simulink model "Robot_calibration_check_Ipos"  (R2021a)
settings: Solver=FixedStepDiscrete  StartTime=0.0  StopTime=tsim  FixedStep=Ts  RelTol=1e-3  EnableMultiTasking=on
InitFcn:
  | Fs = 2048; Ts = 1/Fs;tsim = inf;
undefined symbols (not defined in the file or in its folder): DiscIntNeverNeededParam
libraries: sperte_lib x24, simulink x6, raspberrypiCommlib x2, Quintic_Polynomial_Trajectory_Library x2
(part 1 of 2)
settings Model: SimulationMode=external  Creator=20174295  LastModifiedBy=ghattum
settings SolverCC: AlgebraicLoopSolver=TrustRegion  PositivePriorityOrder=on
settings DataIOCC: SaveOutput=off  DSMLogging=off  SaveTime=off  ReturnWorkspaceOutputs=off
settings OptimizationCC: EnhancedBackFolding=on  PassReuseOutputArgsThreshold=0  MaxStackSize=64  OptimizeBlockOrder=speed  DifferentSizesBufferReuse=on  OptimizationCustomize=off
settings DebuggingCC: InheritedTsInSrcMsg=none  ParameterTunabilityLossMsg=error  SFMachineParentedDataDiag=warning
settings HardwareCC: ProdBitPerPointer=32  ProdBitPerSizeT=32  ProdBitPerPtrDiffT=32  ProdLargestAtomicInteger=Long  ProdLargestAtomicFloat=Double  ProdWordSize=32  ProdLongLongMode=on  ProdHWDeviceType=ARM Compatible->ARM Cortex  UseEmbeddedCoderFeatures=off
settings RTWCC: SystemTargetFile=ert.tlc  HardwareBoard=Raspberry Pi  TLCOptions="-aInlineSetEventsForThisBaseRateFcn=TLC_FALSE -aSuppressMultiTaskScheduler=TLC_FALSE  -aRateBasedStepFcn=0"  TemplateMakefile=ert_default_tmf  PostCodeGenCommand="if (~verLessThan(\"matlab\", \"9.11\")) codertarget.postCodeGenHookCommand(h);  SPERTE_postGenFunc(modelName, buildInfo); else; SPERTE_postGenFunc(h, buildInfo); end"  Toolchain=GNU GCC Embedded Linux  BuildConfiguration=Faster Runs
settings CodeAppCC: ForceParamTrailComments=on  OperatorAnnotations=on
settings ERTTargetCC: ERTCustomFileBanners=off  SupportContinuousTime=on  SupportNonInlinedSFcns=on  RemoveResetFunc=off  SupportVariableSizeSignals=on  ModelStepFunctionPrototypeControlCompliant=off  ExtMode=on  ExtModeStaticAlloc=on  ExtModeMexArgs='10.55.0.1' 0 17726  ERTSrcFileBannerTemplate=codertarget_code_template.cgt  ERTHdrFileBannerTemplate=codertarget_code_template.cgt  ERTDataSrcFileTemplate=codertarget_code_template.cgt  ERTDataHdrFileTemplate=codertarget_code_template.cgt

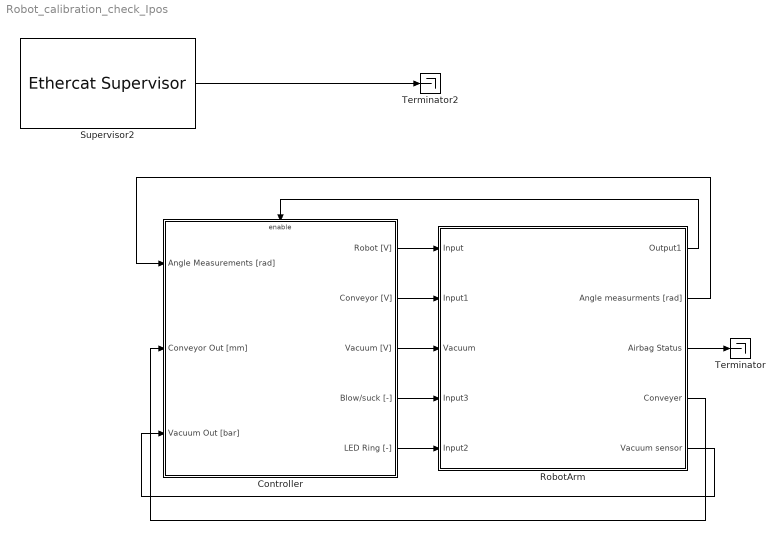
== system Robot_calibration_check_Ipos ==
  Controller : Subsystem
  RobotArm : Subsystem
      mask help:
      | Robot Arm
      | Hardware: Brom Mechatronica
      | Software: Bob Bindels, Victor Dolk, Quinten Swaan, Hugo Thelosen
      mask Display:
      | image(imread('picture_robot.jpg'))
      | color('red');port_label('output', 1, 'Homing Busy [-]')
      | port_label('output', 2, 'Angle Measurements [rad]')
      | port_label('output', 3, 'Airbag Status [-]')
      | port_label('output', 4, 'Conveyor Belt [mm]')
      | port_label('output', 5, 'Vacuum Sensor [bar]')
      | port_label('input', 1, 'Input Robot [V]')
      | port_label('input', 2,'Input Conv [V]' )
      | port_label('input', 3,'Input Vac [V]' )
      | port_label('input', 4,'IO Vac [-]' )
      | port_label('input', 5,'LED-Ring [-]' )
  Supervisor2 : sperte_lib/Ethercat Supervisor  Description=Must be executed first, keep at -1 priority (highest)  Priority=-3  portid=0  ectimeout=500
      settings: SourceProductName=SPERTE project library
  Terminator : Terminator
  Terminator2 : Terminator
  wires:
  Supervisor2/1 -> Terminator2/1
  Controller/1(Robot [V]) -> RobotArm/1(Input)
  RobotArm/1(Output1) -> Controller/Enable
  RobotArm/2(Angle measurments [rad]) -> Controller/1(Angle Measurements [rad])
  Controller/2("Conveyor [V] ") -> RobotArm/2(Input1)
  Controller/3("Vacuum [V] ") -> RobotArm/3(Vacuum)
  Controller/4(Blow/suck [-]) -> RobotArm/4(Input3)
  RobotArm/3(Airbag Status) -> Terminator/1
  RobotArm/4(Conveyer) -> Controller/2(Conveyor Out [mm])
  Controller/5(LED Ring [-]) -> RobotArm/5(Input2)
  RobotArm/5(Vacuum sensor) -> Controller/3(Vacuum Out [bar])

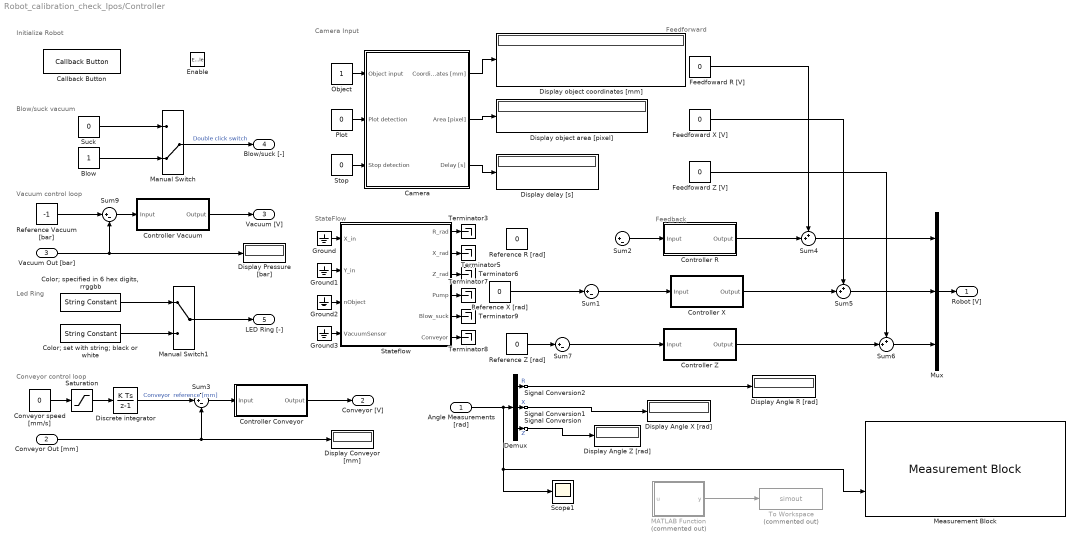
== system Robot_calibration_check_Ipos/Controller ==
  note: Feedforward
  note: StateFlow
  note: Camera Input
  note: Vacuum control loop
  note: Conveyor control loop
  note: Blow/suck vacuum
  note: Led Ring
  note: Feedback
  note: Initialize Robot
  Angle Measurements [rad] : Inport
  Conveyor Out [mm] : Inport  Port=2
  Vacuum Out [bar] : Inport  Port=3
  "Enable " : EnablePort
  " Blow" : Constant
  Callback Button : CallbackButton  ButtonText=INITIALIZE MODEL
      settings: ClickFcn=|
      | robot_number = input('What is your Robot number?: ');
      | file_name_simulink = get_param(bdroot, 'Name');
      | load('calibration_matrix.mat');
      | [camera_calibration_x_pixels,camera_calibration_y_pixels,camera_calibration_pixels_per_mm,camera_calibration_ROI,robot_calibration_r,robot_calibration_x, robot_calibration_z] = Calibrate_Robot_Settings(robot_number,calibration)
      | 
      | set_param(file_name_simulink+"/RobotArm/Supervisor/set_robot_calibration_r",'Value',num2str(robot_calibration_r));
      | set_param(file_name_simulink+"/RobotArm/Supervisor/set_robot_calibration_x",'Value',num2str(robot_calibration_x));
      | set_param(file_name_simulink+"/RobotArm/Supervisor/set_robot_calibration_z",'Value',num2str(robot_calibration_z));
      | 
      | % robot_calibration_r = eval(get_param(file_name_simulink+"/RobotArm/Supervisor/set_robot_calibration_r",'Value'));
      | % robot_calibration_x = eval(get_param(file_name_simulink+"/RobotArm/Supervisor/set_robot_calibration_x",'Value'));
      | % robot_calibration_z = eval(get_param(file_name_simulink+"/RobotArm/Supervisor/set_robot_calibration_z",'Value'));
      | 
      | clear calibration
      | msgbox('Successfully initialized the model.');
  Camera : Subsystem
  Color; set with string; black or white : StringConstant  String='black'
  "Color; specified in 6 hex digits, rrggbb" : StringConstant  String='0072bd'
  Controller Conveyor : Subsystem
  Controller R : Subsystem
  Controller Vacuum : Subsystem
  Controller X : Subsystem
  Controller Z : Subsystem
  Conveyor speed [mm/s] : Constant  Value=0
  Demux : Demux  Outputs=3
  Discrete integrator : DiscreteIntegrator  SampleTime=-1  ICPrevOutput=DiscIntNeverNeededParam  ICPrevScaledInput=DiscIntNeverNeededParam
  Display Angle R [rad] : Display
  Display Angle X [rad] : Display
  Display Angle Z [rad] : Display
  Display Conveyor [mm] : Display
  Display Pressure [bar] : Display
  Display delay [s] : Display
  Display object area [pixel] : Display
  Display object coordinates [mm] : Display
  Feedfoward R [V] : Constant  Value=0
  Feedfoward X [V] : Constant  Value=0
  Feedfoward Z [V] : Constant  Value=0
  Ground{,1..3} (4 alike) : Ground
  MATLAB Function : MATLAB Function  Commented=on  TreatAsAtomicUnit=on
  Manual Switch : ManualSwitch  CurrentSetting=0
  Manual Switch1 : ManualSwitch
  Measurement Block : sperte_lib/Measurement Block  Description=|  Priority=-1  N_samples=1  triggertype=1  trigger_command=0
      | Perform on-demand measurements to file using this block.
      | 
      | It can be used in 2 ways:
      | 1) Set the mask triggertype parameter to manual and use the trigger input signal to trigger a measurement.
      | You can do this by providing a 0 to 1 transition.
      | Keep it low after you start/complete the measurement, or it will measure again.
      | A file is created with measurement_0,1,2... etc
      | 
      | 2) Keep the model running, and trigger a measurement from the commandline or Matlab script.
      | For example:
      | 
      | % How many samples to measure?
      | N_samples = Fs*5;
      | % Do the measurement
      | SPERTE_Perform_Measurement(N_samples);
      | % Get the latest file
      | file_list = SPERTE_Get_Latest_Measurement(p,1,'./data');
      | % How many signals did you record?
      | N_signals = 3;
      | % Convert the .bin to .mat and return the results
      | measurement = SPERTE_Bin_To_Mat(file_list,N_signals);
      settings: SourceProductName=SPERTE project library
  Mux : Mux  Inputs=3
  Object : Constant
  Plot : Constant  Value=0
  Reference Vacuum [bar] : Constant  Value=-1
  Reference R [rad] : Constant  Value=0
  Reference X [rad] : Constant  Value=0
  Reference Z [rad] : Constant  Value=0
  "Saturation " : Saturate  UpperLimit=100  LowerLimit=-100
  Scope1 : Scope
  Signal Conversion : SignalConversion  OverrideOpt=off
  Signal Conversion1 : SignalConversion  OverrideOpt=off
  Signal Conversion2 : SignalConversion  OverrideOpt=off
  "Stateflow " : Stateflow chart  TreatAsAtomicUnit=on
  Stop : Constant  Value=0
  Suck : Constant  Value=0
  Sum{1..3,7,9} (5 alike) : Sum  Inputs=|+-
  Sum4 : Sum  Inputs=++|  InputSameDT=on  SaturateOnIntegerOverflow=on  OutDataTypeStr=Inherit: Same as first input
  Sum5 : Sum  Inputs=++|  InputSameDT=on  SaturateOnIntegerOverflow=on  OutDataTypeStr=Inherit: Same as first input
  Sum6 : Sum  Inputs=++|  InputSameDT=on  SaturateOnIntegerOverflow=on  OutDataTypeStr=Inherit: Same as first input
  Terminator{3,5..9} (6 alike) : Terminator
  To Workspace : ToWorkspace  Commented=on  VariableName=simout  SaveFormat=Timeseries  SampleTime=-1
  Robot [V] : Outport
  "Conveyor [V] " : Outport  Port=2
  "Vacuum [V] " : Outport  Port=3
  Blow/suck [-] : Outport  Port=4
  LED Ring [-] : Outport  Port=5
  wires:
  Manual Switch/1 -> Blow/suck [-]/1  "Double click switch"
  Suck/1 -> Manual Switch/1
  " Blow"/1 -> Manual Switch/2
  Feedfoward Z [V]/1 -> Sum6/1
  Sum7/1 -> Controller Z/1(Input)
  Controller Z/1(Output) -> Sum6/2
  Controller X/1(Output) -> Sum5/2
  Controller R/1(Output) -> Sum4/2
  Demux/2 -> Signal Conversion1/1  "X"
  Mux/1 -> Robot [V]/1
  Demux/3 -> Signal Conversion/1  "Z"
  Angle Measurements [rad]/1 -> Measurement Block/2, Scope1/1, Demux/1
  "Color; specified in 6 hex digits, rrggbb"/1 -> Manual Switch1/1
  Color; set with string; black or white/1 -> Manual Switch1/2
  Demux/1 -> Signal Conversion2/1  "R"
  Manual Switch1/1 -> LED Ring [-]/1
  Vacuum Out [bar]/1 -> Sum9/2, Display Pressure [bar]/1
  Sum1/1 -> Controller X/1(Input)
  Stop/1 -> Camera/3(Stop detection)
  Object/1 -> Camera/1(Object input)
  Plot/1 -> Camera/2(Plot detection)
  Reference Vacuum [bar]/1 -> Sum9/1
  Sum9/1 -> Controller Vacuum/1(Input)
  Controller Vacuum/1(Output) -> "Vacuum [V] "/1
  Signal Conversion/1 -> Display Angle Z [rad]/1
  Signal Conversion1/1 -> Display Angle X [rad]/1
  Signal Conversion2/1 -> Display Angle R [rad]/1
  Ground/1 -> "Stateflow "/1(X_in)
  Ground1/1 -> "Stateflow "/2(Y_in)
  Ground2/1 -> "Stateflow "/3(nObject)
  Ground3/1 -> "Stateflow "/4(VacuumSensor)
  "Stateflow "/1(R_rad) -> Terminator3/1
  "Stateflow "/2(X_rad) -> Terminator5/1
  "Stateflow "/3(Z_rad) -> Terminator6/1
  "Stateflow "/4(Pump) -> Terminator7/1
  "Stateflow "/5(Blow_suck) -> Terminator9/1
  "Stateflow "/6(Conveyor) -> Terminator8/1
  Discrete integrator/1 -> Sum3/1  "Conveyor  reference [mm]"
  Conveyor speed [mm/s]/1 -> "Saturation "/1
  "Saturation "/1 -> Discrete integrator/1
  Camera/1(Coordinates [mm]) -> Display object coordinates [mm]/1
  Camera/3(Delay [s]) -> Display delay [s]/1
  Camera/2(Area [pixel]) -> Display object area [pixel]/1
  Sum6/1 -> Mux/3
  Controller Conveyor/1(Output) -> "Conveyor [V] "/1
  Sum4/1 -> Mux/1
  Sum2/1 -> Controller R/1(Input)
  Reference Z [rad]/1 -> Sum7/1
  Feedfoward X [V]/1 -> Sum5/1
  Sum5/1 -> Mux/2
  Reference X [rad]/1 -> Sum1/1
  Feedfoward R [V]/1 -> Sum4/1
  Conveyor Out [mm]/1 -> Display Conveyor [mm]/1, Sum3/2
  Sum3/1 -> Controller Conveyor/1(Input)
  MATLAB Function/1(y) -> To Workspace/1

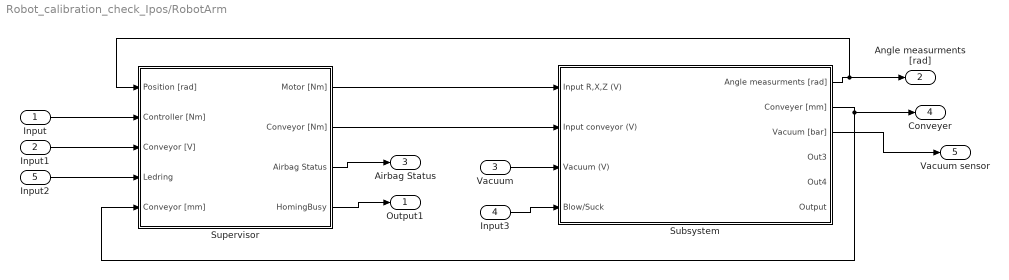
== system Robot_calibration_check_Ipos/RobotArm ==
  Input : Inport
  Input1 : Inport  Port=2
  Vacuum : Inport  Port=3
  Input3 : Inport  Port=4
  Input2 : Inport  Port=5
  Subsystem : Subsystem
  Supervisor : Subsystem
  Output1 : Outport
  Angle measurments [rad] : Outport  Port=2
  Airbag Status : Outport  Port=3
  Conveyer : Outport  Port=4
  Vacuum sensor : Outport  Port=5
  wires:
  Supervisor/1(Motor [Nm]) -> Subsystem/1(Input R,X,Z (V))
  Subsystem/2(Conveyer [mm]) -> Supervisor/5(Conveyor [mm]), Conveyer/1
  Supervisor/4(HomingBusy) -> Output1/1
  Input/1 -> Supervisor/2(Controller [Nm])
  Subsystem/1(Angle measurments [rad]) -> Supervisor/1(Position [rad]), Angle measurments [rad]/1
  Input1/1 -> Supervisor/3(Conveyor [V])
  Input3/1 -> Subsystem/4(Blow/Suck)
  Supervisor/3(Airbag Status) -> Airbag Status/1
  Supervisor/2(Conveyor [Nm]) -> Subsystem/2(Input conveyor (V))
  Input2/1 -> Supervisor/4(Ledring)
  Subsystem/3(Vacuum [bar]) -> Vacuum sensor/1
  Vacuum/1 -> Subsystem/3(Vacuum (V))

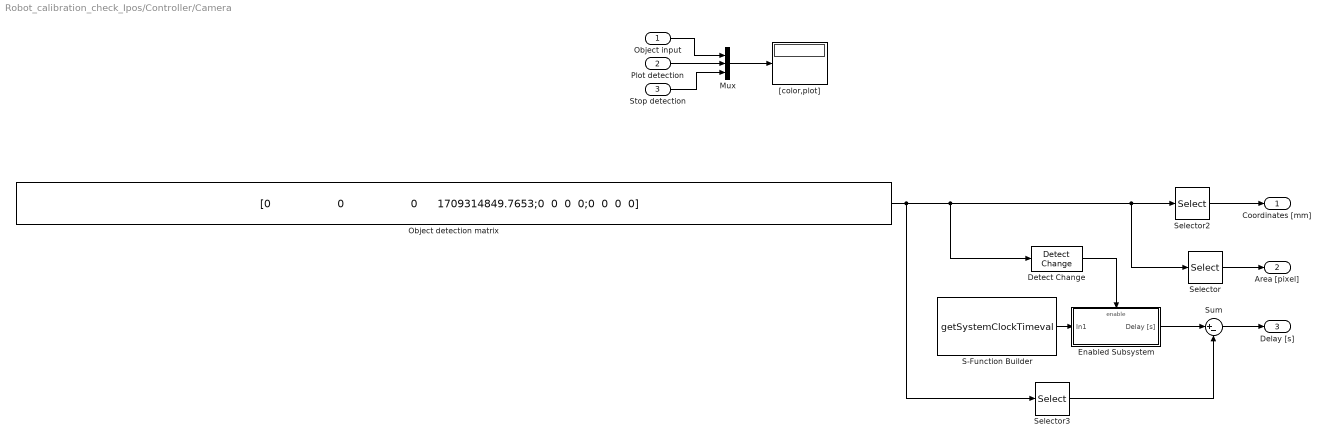
== system Robot_calibration_check_Ipos/Controller/Camera ==
  Object input : Inport
  Plot detection : Inport  Port=2
  Stop detection : Inport  Port=3
  Detect Change : simulink/Logic and Bit Operations/Detect Change  vinit=0  OutDataTypeStr=boolean
  Enabled Subsystem : Subsystem  TreatAsAtomicUnit=on
  Mux : Mux  Inputs=3
  Object detection matrix : Constant  Value="[0                    0                    0      1709314849.7653;0  0  0  0;0  0  0  0]"  VectorParams1D=off
  S-Function Builder : S-Function  InitFcn=try, set_param(gcb,'FunctionName','getSystemClockTimeval'), end  FunctionName=getSystemClockTimeval  SFunctionModules=getSystemClockTimeval_wrapper  SFunctionDeploymentMode=off  EnableBusSupport=off  mask(S-Function Builder){}
      mask help: Simulink:masks:SFunctionBuilder_MD
      mask init:
      | val = [[.9  0.75 0.75 1 1 .9 .9 1]',[1 1 0.75 0.75 .9 .9 1 .9]'];try , sys = get_param(gcb,'SfunBuilderFcnName');if isempty(sys), sys = get_param(gcb,'FunctionName'); end,catch, sys = get_param(gcb,'FunctionName'); end
      settings: CopyFcn=set_param(gcbh,'LinkStatus','none')  PreSaveFcn=try, set_param(gcb,'FunctionName','getSystemClockTimeval'), end  OpenFcn=sfunctionwizard(gcbh)
      mask Display: plot(val(:,1),val(:,2)),disp(sys),port_label('output',1,'y2')
  Selector : Selector  NumberOfDimensions=2  InputPortWidth=3  IndexOptions=Index vector (dialog),Index vector (dialog)  Indices=[3],[1:3]  OutputSizes=1,1
  Selector2 : Selector  NumberOfDimensions=2  InputPortWidth=3  IndexOptions=Select all,Index vector (dialog)  Indices=1,[1:3]  OutputSizes=1,1
  Selector3 : Selector  NumberOfDimensions=2  InputPortWidth=3  IndexOptions=Index vector (dialog),Index vector (dialog)  Indices=1,4  OutputSizes=1,1
  Sum : Sum  Inputs=|+-
  "[color,plot]" : Display
  Coordinates [mm] : Outport
  Area [pixel] : Outport  Port=2
  Delay [s] : Outport  Port=3
  wires:
  Object input/1 -> Mux/1
  Plot detection/1 -> Mux/2
  Mux/1 -> "[color,plot]"/1
  Stop detection/1 -> Mux/3
  Selector2/1 -> Coordinates [mm]/1
  Object detection matrix/1 -> Selector3/1, Detect Change/1, Selector/1, Selector2/1
  Detect Change/1 -> Enabled Subsystem/Enable
  S-Function Builder/1 -> Enabled Subsystem/1(In1)
  Enabled Subsystem/1(Delay [s]) -> Sum/1
  Sum/1 -> Delay [s]/1
  Selector3/1 -> Sum/2
  Selector/1 -> Area [pixel]/1

== system Robot_calibration_check_Ipos/Controller/Controller Conveyor ==
  Input : Inport
  Dct1lowpass : sperte_lib/Dct1lowpass  f_den=40
      settings: SourceProductName=SPERTE project library
  Dctintegrator3 : S-Function  FunctionName=dweakint  Parameters=f_num, 0.001  SFunctionDeploymentMode=off  EnableBusSupport=off  mask(dctools){f_num=0.05}
      mask prompts: f_num "Zero [Hz]"
      mask help: This block implements a discrete time weak integrator filter.
      mask Display: disp('DCT integrator')
  Dctleadlag : sperte_lib/Dctleadlag  f_num=3  f_den=30
      settings: SourceProductName=SPERTE project library
  Gain1 : Gain  Gain=0.05
  Output : Outport
  wires:
  Input/1 -> Gain1/1
  Dctintegrator3/1 -> Dct1lowpass/1
  Dctleadlag/1 -> Output/1
  Gain1/1 -> Dctintegrator3/1
  Dct1lowpass/1 -> Dctleadlag/1

== system Robot_calibration_check_Ipos/Controller/Controller R ==
  Input : Inport
  Gain : Gain  Gain=5
  Output : Outport
  wires:
  Input/1 -> Gain/1
  Gain/1 -> Output/1

== system Robot_calibration_check_Ipos/Controller/Controller Vacuum ==
  Input : Inport
  Gain1 : Gain  Gain=-10
  Output : Outport
  wires:
  Input/1 -> Gain1/1
  Gain1/1 -> Output/1

== system Robot_calibration_check_Ipos/Controller/Controller X ==
  Input : Inport
  Gain1 : Gain  Gain=5
  Output : Outport
  wires:
  Gain1/1 -> Output/1
  Input/1 -> Gain1/1

== system Robot_calibration_check_Ipos/Controller/Controller Z ==
  Input : Inport
  Gain : Gain  Gain=5
  Output : Outport
  wires:
  Input/1 -> Gain/1
  Gain/1 -> Output/1

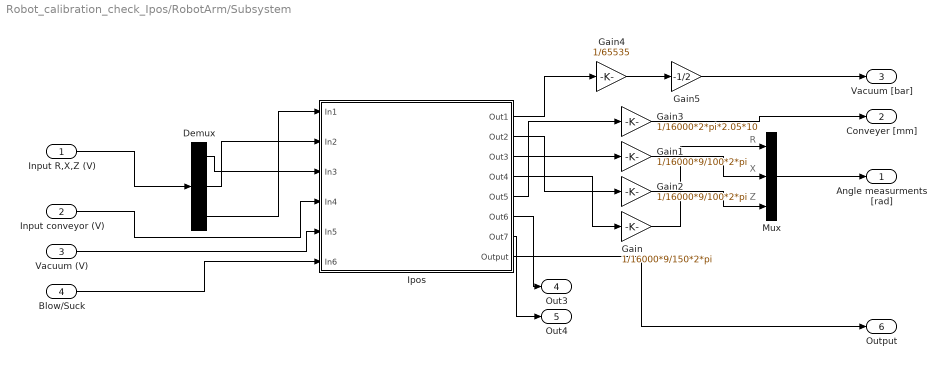
== system Robot_calibration_check_Ipos/RobotArm/Subsystem ==
  note: R
  note: X
  note: Z
  Input R,X,Z (V) : Inport
  Input conveyor (V) : Inport  Port=2
  Vacuum (V) : Inport  Port=3
  Blow/Suck : Inport  Port=4
  Demux : Demux  Outputs=3
  Gain : Gain  Gain=1/16000*9/150*2*pi
  Gain1 : Gain  Gain=1/16000*9/100*2*pi
  Gain2 : Gain  Gain=1/16000*9/100*2*pi
  Gain3 : Gain  Gain=1/16000*2*pi*2.05*10
  Gain4 : Gain  Gain=1/65535
  Gain5 : Gain  Gain=-1/2
  Ipos : Subsystem  mask{link_id=1}
      mask prompts: link_id "Link ID of the specific Ipos"
      mask Display:
      | image('ipos360.JPG'); % Use "Edit Image" on toolstrip to change.
      | port_label('output',1,'ADC')
      | port_label('output',2,'ENC1')
      | port_label('output',3,'ENC2')
      | port_label('output',4,'ENC3')
      | port_label('output',5,'ENC4')
      | port_label('output',6,'DI_t')
      | port_label('output',7,'DI_stop')
      | port_label('input',1,'Torque Conveyor')
      | port_label('input',2,'Torque X')
      | port_label('input',3,'Torque Z')
      | port_label('input',4,'Torque R')
      | port_label('input',5,'Do')
      | port_label('input',6,'setpoint_P')
  Mux : Mux  Inputs=3
  Angle measurments [rad] : Outport
  Conveyer [mm] : Outport  Port=2
  Vacuum [bar] : Outport  Port=3
  Out3 : Outport  Port=4
  Out4 : Outport  Port=5
  Output : Outport  Port=6
  wires:
  Mux/1 -> Angle measurments [rad]/1
  Input conveyor (V)/1 -> Ipos/4(In4)
  Ipos/8(Output) -> Output/1
  Gain1/1 -> Mux/2
  Input R,X,Z (V)/1 -> Demux/1
  Gain/1 -> Mux/1
  Ipos/7(Out7) -> Out4/1
  Gain2/1 -> Mux/3
  Gain3/1 -> Conveyer [mm]/1
  Ipos/1(Out1) -> Gain4/1
  Ipos/6(Out6) -> Out3/1
  Ipos/2(Out2) -> Gain2/1
  Ipos/3(Out3) -> Gain1/1
  Ipos/4(Out4) -> Gain/1
  Ipos/5(Out5) -> Gain3/1
  Demux/2 -> Ipos/2(In2)
  Demux/3 -> Ipos/1(In1)
  Blow/Suck/1 -> Ipos/6(In6)
  Vacuum (V)/1 -> Ipos/5(In5)
  Demux/1 -> Ipos/3(In3)
  Gain4/1 -> Gain5/1
  Gain5/1 -> Vacuum [bar]/1

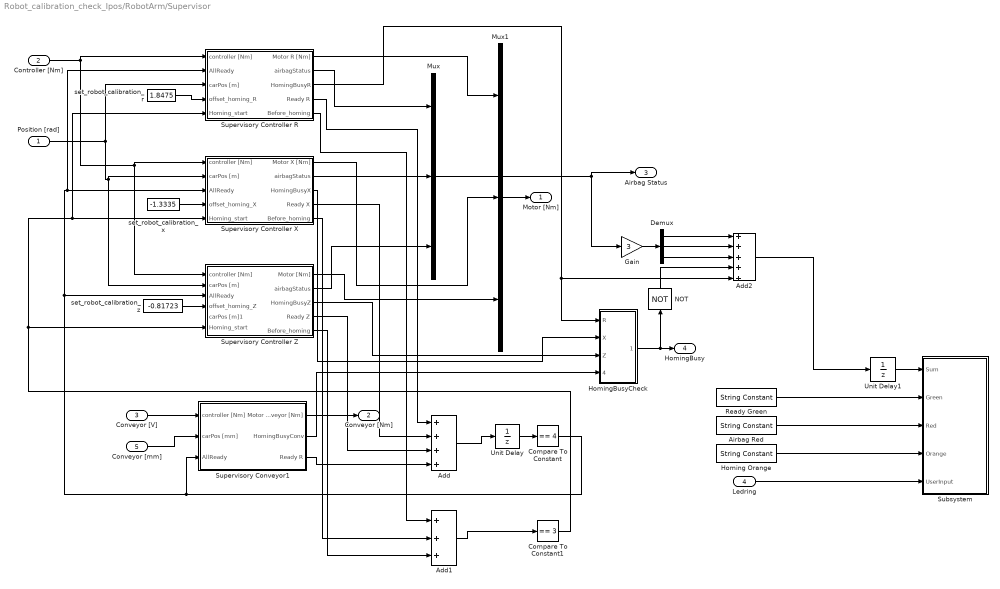
== system Robot_calibration_check_Ipos/RobotArm/Supervisor ==
  Position [rad] : Inport
  Controller [Nm] : Inport  Port=2
  Conveyor [V] : Inport  Port=3
  Ledring : Inport  Port=4
  Conveyor [mm] : Inport  Port=5
  Add : Sum  Inputs=++++
  Add1 : Sum  Inputs=+++
  Add2 : Sum  Inputs=+++++
  Airbag Red : StringConstant  String='00FF0000'
  Compare To Constant : simulink/Logic and Bit Operations/Compare To Constant  relop===  const=4  OutDataTypeStr=boolean
  Compare To Constant1 : simulink/Logic and Bit Operations/Compare To Constant  relop===  const=3  OutDataTypeStr=boolean
  Demux : Demux  Outputs=3
  Gain : Gain  Gain=3
  Homing Orange : StringConstant  String='00FF3900'
  HomingBusyCheck : Subsystem
  Mux : Mux  Inputs=3
  Mux1 : Mux  Inputs=3
  NOT : Logic  Operator=NOT  IconShape=distinctive  AllPortsSameDT=off  OutDataTypeStr=boolean
  Ready Green : StringConstant  String='0000FF00'
  Subsystem : Subsystem
  Supervisory Controller R : Subsystem
  Supervisory Controller X : Subsystem
  Supervisory Controller Z : Subsystem
  Supervisory Conveyor1 : Subsystem
  Unit Delay : UnitDelay  SampleTime=-1  HasFrameUpgradeWarning=on
  Unit Delay1 : UnitDelay  SampleTime=-1  HasFrameUpgradeWarning=on
  set_robot_calibration_r : Constant  Value=1.8475
  set_robot_calibration_x : Constant  Value=-1.3335
  set_robot_calibration_z : Constant  Value=-0.81723
  Motor [Nm] : Outport
  Conveyor [Nm] : Outport  Port=2
  Airbag Status : Outport  Port=3
  HomingBusy : Outport  Port=4
  wires:
  Controller [Nm]/1 -> Supervisory Controller R/1(controller [Nm]), Supervisory Controller X/1(controller [Nm]), Supervisory Controller Z/1(controller [Nm])
  Supervisory Controller R/2(airbagStatus) -> Mux/1
  Supervisory Controller X/2(airbagStatus) -> Mux/2
  Supervisory Controller Z/2(airbagStatus) -> Mux/3
  Position [rad]/1 -> Supervisory Controller R/3(carPos [m]), Supervisory Controller X/2(carPos [m]), Supervisory Controller Z/2(carPos [m])
  Mux1/1 -> Motor [Nm]/1
  Supervisory Controller X/3(HomingBusyX) -> HomingBusyCheck/2(X)
  Supervisory Controller Z/3(HomingBusyZ) -> HomingBusyCheck/3(Z)
  HomingBusyCheck/1(Out1) -> NOT/1, HomingBusy/1
  Supervisory Controller R/4(Ready R) -> Add/1
  Supervisory Controller X/4(Ready X) -> Add/2
  Supervisory Controller Z/4(Ready Z) -> Add/3
  Compare To Constant/1 -> Supervisory Controller X/3(AllReady), Supervisory Controller R/2(AllReady), Supervisory Controller Z/3(AllReady), Supervisory Conveyor1/3(AllReady)
  Add/1 -> Unit Delay/1
  Unit Delay/1 -> Compare To Constant/1
  set_robot_calibration_r/1 -> Supervisory Controller R/4(offset_homing_R)
  set_robot_calibration_x/1 -> Supervisory Controller X/4(offset_homing_X)
  set_robot_calibration_z/1 -> Supervisory Controller Z/4(offset_homing_Z)
  Mux/1 -> Airbag Status/1, Gain/1
  Supervisory Controller R/5(Before_homing) -> Add1/1
  Supervisory Controller X/5(Before_homing) -> Add1/2
  Supervisory Controller Z/5(Before_homing) -> Add1/3
  Add1/1 -> Compare To Constant1/1
  Compare To Constant1/1 -> Supervisory Controller Z/6(Homing_start), Supervisory Controller X/5(Homing_start), Supervisory Controller R/5(Homing_start)
  Supervisory Controller R/1(Motor R [Nm]) -> Mux1/1
  Conveyor [V]/1 -> Supervisory Conveyor1/1(controller [Nm])
  Supervisory Conveyor1/3(Ready R) -> Add/4
  Supervisory Conveyor1/2(HomingBusyConv) -> HomingBusyCheck/4(Conv)
  Conveyor [mm]/1 -> Supervisory Conveyor1/2(carPos [mm])
  Add2/1 -> Unit Delay1/1
  Ledring/1 -> Subsystem/5(UserInput)
  Gain/1 -> Demux/1
  Airbag Red/1 -> Subsystem/3(Red)
  Ready Green/1 -> Subsystem/2(Green)
  Homing Orange/1 -> Subsystem/4(Orange)
  Unit Delay1/1 -> Subsystem/1(Sum)
  Supervisory Controller R/3(HomingBusyR) -> Add2/5, HomingBusyCheck/1(R)
  NOT/1 -> Add2/4
  Demux/2 -> Add2/2
  Demux/3 -> Add2/3
  Demux/1 -> Add2/1
  Supervisory Controller X/1(Motor X [Nm]) -> Mux1/2
  Supervisory Controller Z/1(Motor [Nm]) -> Mux1/3
  Supervisory Conveyor1/1(Motor Conveyor [Nm]) -> Conveyor [Nm]/1

== system Robot_calibration_check_Ipos/Controller/Camera/Enabled Subsystem ==
  In1 : Inport
  Enable : EnablePort
  Delay [s] : Outport
  wires:
  In1/1 -> Delay [s]/1

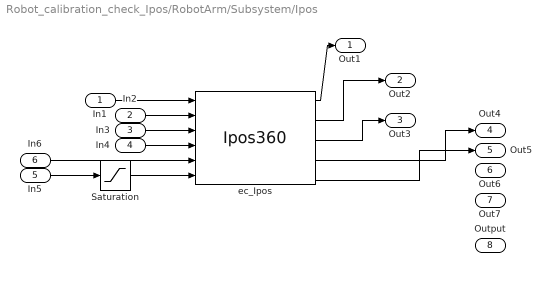
== system Robot_calibration_check_Ipos/RobotArm/Subsystem/Ipos ==
  In1 : Inport
  In2 : Inport  Port=2
  In3 : Inport  Port=3
  In4 : Inport  Port=4
  In5 : Inport  Port=5
  In6 : Inport  Port=6
  Saturation : Saturate  UpperLimit=255  LowerLimit=0
  ec_Ipos : S-Function  FunctionName=Ipos360  Parameters=link_id  SFunctionDeploymentMode=off  EnableBusSupport=off  mask{link_id=link_id}
      mask prompts: link_id "link_id >= 0"
      mask Display:
      | port_label('output',1,'ADC')
      | port_label('output',2,'ENC Z')
      | port_label('output',3,'ENC X')
      | port_label('output',4,'ENC R')
      | port_label('output',5,'ENC C')
      | port_label('output',6,'DI_t')
      | port_label('output',7,'DI_stop')
      | % port_label('output',8,'ENC5')
      | port_label('input',1,'`Torque Z')
      | port_label('input',2,'Torque X')
      | port_label('input',3,'Torque R')
      | port_label('input',4,'Torque C')
      | port_label('input',5,'Do')
      | port_label('input',6,'setpoint_P')
  Out1 : Outport
  Out2 : Outport  Port=2
  Out3 : Outport  Port=3
  Out4 : Outport  Port=4
  Out5 : Outport  Port=5
  Out6 : Outport  Port=6
  Out7 : Outport  Port=7
  Output : Outport  Port=8
  wires:
  ec_Ipos/5 -> Out5/1
  ? -> Out7/1
  ec_Ipos/4 -> Out4/1
  ec_Ipos/3 -> Out3/1
  ec_Ipos/1 -> Out1/1
  ec_Ipos/2 -> Out2/1
  ? -> Out6/1
  ? -> Output/1
  In2/1 -> ec_Ipos/2
  In3/1 -> ec_Ipos/3
  In4/1 -> ec_Ipos/4
  In1/1 -> ec_Ipos/1
  In5/1 -> Saturation/1
  In6/1 -> ec_Ipos/5
  Saturation/1 -> ec_Ipos/6

== system Robot_calibration_check_Ipos/RobotArm/Supervisor/HomingBusyCheck ==
  R : Inport
  X : Inport  Port=2
  Z : Inport  Port=3
  Conv : Inport  Port=4
  Add : Sum  Inputs=++++
  Add1 : Sum  Inputs=+-
  Constant : Constant
  Sign : Signum
  Out1 : Outport
  wires:
  Add/1 -> Sign/1
  R/1 -> Add/1
  X/1 -> Add/2
  Z/1 -> Add/3
  Constant/1 -> Add1/1
  Sign/1 -> Add1/2
  Add1/1 -> Out1/1
  Conv/1 -> Add/4

== system Robot_calibration_check_Ipos/RobotArm/Supervisor/Subsystem ==
  Sum : Inport
  Green : Inport  Port=2
  Red : Inport  Port=3
  Orange : Inport  Port=4
  UserInput : Inport  Port=5
  Homing Running Switch : Switch  Threshold=0.5
  Homing Running Switch1 : Switch  Threshold=2.5
  Homing Running Switch2 : Switch  Threshold=50
  LED Ring : Subsystem
  wires:
  Homing Running Switch/1 -> LED Ring/1(U)
  Green/1 -> Homing Running Switch2/1
  UserInput/1 -> Homing Running Switch/3
  Homing Running Switch1/1 -> Homing Running Switch/1
  Red/1 -> Homing Running Switch2/3
  Orange/1 -> Homing Running Switch1/3
  Sum/1 -> Homing Running Switch2/2, Homing Running Switch1/2, Homing Running Switch/2
  Homing Running Switch2/1 -> Homing Running Switch1/1

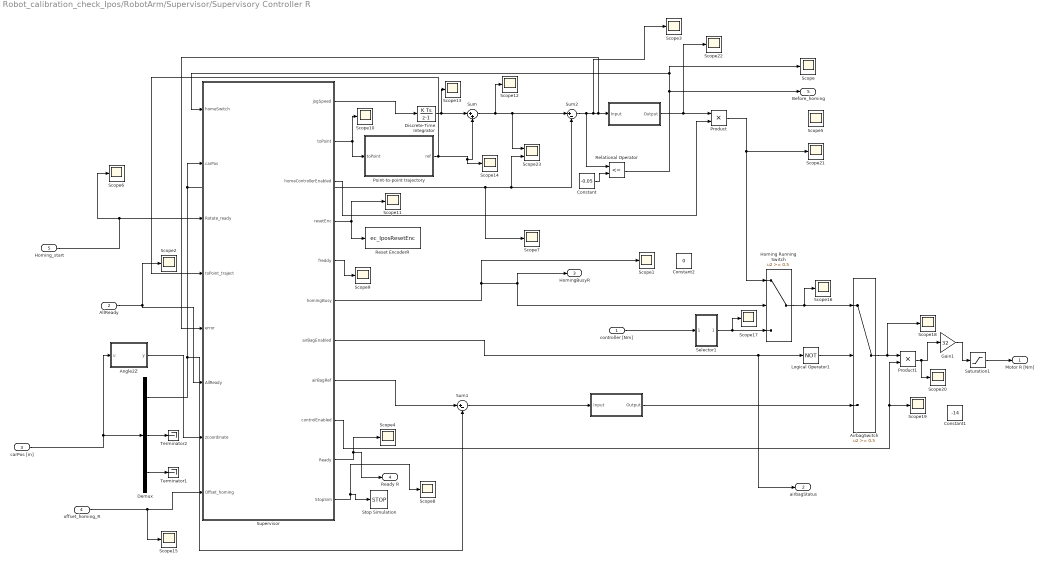
== system Robot_calibration_check_Ipos/RobotArm/Supervisor/Supervisory Controller R ==
  controller [Nm] : Inport
  AllReady : Inport  Port=2
  carPos [m] : Inport  Port=3
  offset_homing_R : Inport  Port=4
  Homing_start : Inport  Port=5
  " " : Subsystem
  "   " : Subsystem
  AirbagSwitch : Switch  Threshold=0.5
  Angle2Z : MATLAB Function  TreatAsAtomicUnit=on
  Constant : Constant  Value=-0.05
  Constant1 : Constant  Value=-14
  Constant2 : Constant  Value=0
  Demux : Demux  Outputs=3
  Discrete-Time Integrator : DiscreteIntegrator  SampleTime=-1  ICPrevOutput=DiscIntNeverNeededParam  ICPrevScaledInput=DiscIntNeverNeededParam
  Gain1 : Gain  Gain=32
  Homing Running Switch : Switch  Threshold=0.5
  Logical Operator1 : Logic  Operator=NOT  AllPortsSameDT=off  OutDataTypeStr=boolean
  Point-to-point trajectory : Subsystem
  Product : Product  RndMeth=Zero
  Product1 : Product  RndMeth=Zero
  Relational Operator : RelationalOperator  Operator=<=  OutDataTypeStr=boolean  RndMeth=Nearest
  Reset EncoderR : S-Function  FunctionName=ec_IposResetEnc  Parameters=ipos_id  SFunctionDeploymentMode=off  EnableBusSupport=off  mask{ipos_id=3}
      mask prompts: ipos_id "Ipos ID (from 0 till 3)"
  Saturation1 : Saturate  UpperLimit=127  LowerLimit=-127
  Scope{,1..22} (23 alike) : Scope
  Scope23 : Scope  NumInputPorts=2
  Selector1 : Subsystem
  Stop Simulation : Stop
  Sum : Sum  Inputs=|++
  Sum1 : Sum  Inputs=|+-
  Sum2 : Sum  Inputs=|+-
  Supervisor : Stateflow chart  TreatAsAtomicUnit=on
  Terminator1 : Terminator
  Terminator2 : Terminator
  Motor R [Nm] : Outport
  airbagStatus : Outport  Port=2
  HomingBusyR : Outport  Port=3
  Ready R : Outport  Port=4
  Before_homing : Outport  Port=5
  wires:
  Homing Running Switch/1 -> Scope16/1, AirbagSwitch/1
  Relational Operator/1 -> Scope/1, Supervisor/1(homeSwitch), Before_homing/1
  Point-to-point trajectory/1(ref) -> Sum/2, Scope14/1, Supervisor/4(toPoint_traject)
  Supervisor/6(homingBusy) -> Scope1/1, Homing Running Switch/2, HomingBusyR/1
  Supervisor/3(homeControllerEnabled) -> Product/2
  Supervisor/2(toPoint) -> Point-to-point trajectory/1(toPoint), Scope10/1
  Supervisor/4(resetEnc) -> Reset EncoderR/1, Scope11/1
  Logical Operator1/1 -> AirbagSwitch/2
  Supervisor/8(airBagRef) -> Sum1/1
  AirbagSwitch/1 -> Scope18/1, Product1/1
  Supervisor/9(controlEnabled) -> Product1/2, Scope19/1
  Supervisor/7(airBagEnabled) -> airbagStatus/1, Logical Operator1/1
  Demux/1 -> Sum1/2, Scope23/2, Sum2/2, Scope7/1, Supervisor/2(carPos)
  Demux/2 -> Terminator2/1
  Selector1/1(Out1) -> Scope17/1, Homing Running Switch/3
  carPos [m]/1 -> Demux/1, Angle2Z/1(u)
  Constant/1 -> Relational Operator/2
  Supervisor/10(Ready) -> Scope4/1, Ready R/1
  AllReady/1 -> Scope2/1, Supervisor/6(AllReady)
  Supervisor/11(StopSim) -> Scope8/1, Stop Simulation/1
  Sum2/1 -> Scope3/1, Supervisor/5(error), " "/1(Input), Relational Operator/1
  Demux/3 -> Terminator1/1
  Angle2Z/1(y) -> Supervisor/7(zcoordinate)
  Sum1/1 -> "   "/1(Input)
  "   "/1(Output) -> AirbagSwitch/3
  Discrete-Time Integrator/1 -> Scope13/1, Sum/1
  offset_homing_R/1 -> Scope15/1, Supervisor/8(Offset_homing)
  Supervisor/1(jogSpeed) -> Discrete-Time Integrator/1
  Sum/1 -> Scope12/1, Sum2/1, Scope23/1
  Supervisor/5(freddy) -> Scope9/1
  Homing_start/1 -> Supervisor/3(Rotate_ready), Scope6/1
  controller [Nm]/1 -> Selector1/1(controller [Nm])
  " "/1(Output) -> Scope22/1, Product/1
  Product/1 -> Homing Running Switch/1, Scope21/1
  Gain1/1 -> Saturation1/1
  Product1/1 -> Gain1/1, Scope20/1
  Saturation1/1 -> Motor R [Nm]/1

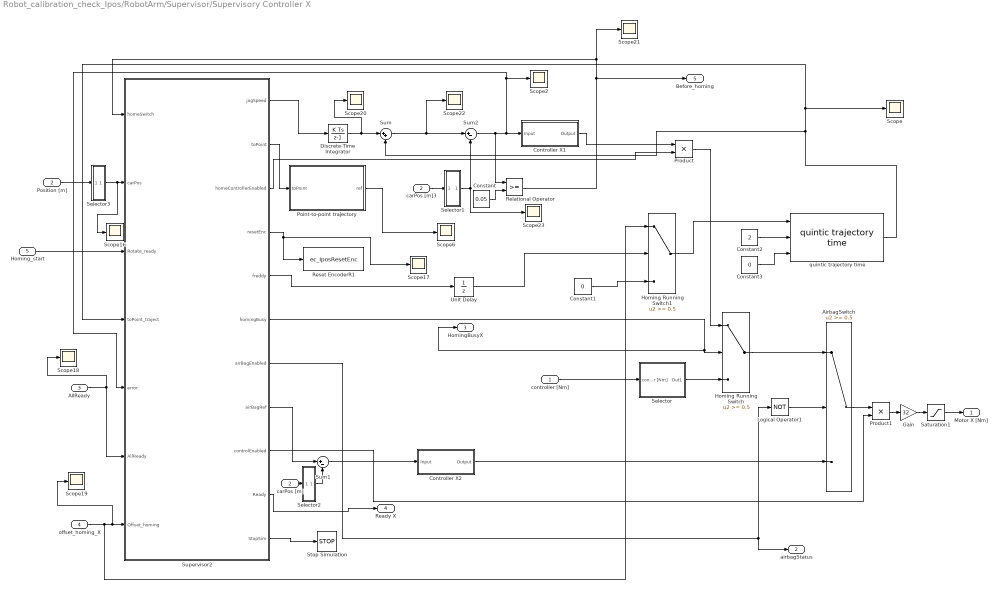
== system Robot_calibration_check_Ipos/RobotArm/Supervisor/Supervisory Controller X ==
  controller [Nm] : Inport
  carPos [m] : Inport  Port=2
  AllReady : Inport  Port=3
  offset_homing_X : Inport  Port=4
  Homing_start : Inport  Port=5
  AirbagSwitch : Switch  Threshold=0.5
  Constant : Constant  Value=0.05
  Constant1 : Constant  Value=0
  Constant2 : Constant  Value=2
  Constant3 : Constant  Value=0
  Controller X1 : Subsystem
  Controller X2 : Subsystem
  Discrete-Time Integrator : DiscreteIntegrator  SampleTime=-1  ICPrevOutput=DiscIntNeverNeededParam  ICPrevScaledInput=DiscIntNeverNeededParam
  Gain : Gain  Gain=32
  Homing Running Switch : Switch  Threshold=0.5
  Homing Running Switch1 : Switch  Threshold=0.5
  Logical Operator1 : Logic  Operator=NOT  AllPortsSameDT=off  OutDataTypeStr=boolean
  Point-to-point trajectory : Subsystem
  Position [m] : InportShadow  Port=2
  Product : Product  RndMeth=Zero
  Product1 : Product  RndMeth=Zero
  Relational Operator : RelationalOperator  OutDataTypeStr=boolean  RndMeth=Nearest
  Reset EncoderR1 : S-Function  FunctionName=ec_IposResetEnc  Parameters=ipos_id  SFunctionDeploymentMode=off  EnableBusSupport=off  mask{ipos_id=1}
      mask prompts: ipos_id "Ipos ID (from 0 till 3)"
  Saturation1 : Saturate  UpperLimit=127  LowerLimit=-127
  Scope{,2,6,16..23} (11 alike) : Scope
  Selector : Subsystem
  Selector1 : Subsystem
  Selector2 : Subsystem
  Selector3 : Subsystem
  Stop Simulation : Stop
  Sum : Sum  Inputs=|++
  Sum1 : Sum  Inputs=|+-
  Sum2 : Sum  Inputs=|+-
  Supervisor2 : Stateflow chart  TreatAsAtomicUnit=on
  Unit Delay : UnitDelay  SampleTime=-1  HasFrameUpgradeWarning=on
  carPos [m]3 : InportShadow  Port=2
  quintic trajectory time : Quintic_Polynomial_Trajectory_Library/quintic trajectory time  SystemSampleTime=-1  VariantActivationTime=update diagram  Latency=0  AutoFrameSizeCalculation=off
      settings: SourceProductName=Robotarm library
  Motor X [Nm] : Outport
  airbagStatus : Outport  Port=2
  HomingBusyX : Outport  Port=3
  Ready X : Outport  Port=4
  Before_homing : Outport  Port=5
  wires:
  Position [m]/1 -> Selector3/1(In1)
  Product1/1 -> Gain/1
  AirbagSwitch/1 -> Product1/1
  carPos [m]/1 -> Selector2/1(In1)
  Sum1/1 -> Controller X2/1(Input)
  Logical Operator1/1 -> AirbagSwitch/2
  carPos [m]3/1 -> Selector1/1(In1)
  Homing Running Switch/1 -> AirbagSwitch/1
  controller [Nm]/1 -> Selector/1(controller [Nm])
  Selector/1(Out1) -> Homing Running Switch/3
  Selector1/1(Out1) -> Sum2/2, Scope23/1
  Selector2/1(Out1) -> Sum1/2
  Constant/1 -> Relational Operator/2
  Controller X2/1(Output) -> AirbagSwitch/3
  Sum2/1 -> Scope2/1, Supervisor2/5(error), Controller X1/1(Input), Relational Operator/1
  Controller X1/1(Output) -> Product/1
  Sum/1 -> Scope22/1, Sum2/1
  Discrete-Time Integrator/1 -> Scope20/1, Sum/1
  Supervisor2/1(jogSpeed) -> Discrete-Time Integrator/1
  Supervisor2/2(toPoint) -> Point-to-point trajectory/1(toPoint)
  Supervisor2/3(homeControllerEnabled) -> Product/2
  Supervisor2/4(resetEnc) -> Reset EncoderR1/1, Scope17/1
  Supervisor2/6(homingBusy) -> Homing Running Switch/2, HomingBusyX/1
  Supervisor2/7(airBagEnabled) -> airbagStatus/1, Logical Operator1/1
  Supervisor2/8(airBagRef) -> Sum1/1
  Supervisor2/9(controlEnabled) -> Product1/2
  Supervisor2/10(Ready) -> Ready X/1
  Supervisor2/11(StopSim) -> Stop Simulation/1
  Selector3/1(carPos) -> Scope16/1, Supervisor2/2(carPos)
  AllReady/1 -> Scope18/1, Supervisor2/6(AllReady)
  offset_homing_X/1 -> Homing Running Switch1/1, Scope19/1, Supervisor2/7(Offset_homing)
  Point-to-point trajectory/1(ref) -> Scope6/1
  Relational Operator/1 -> Before_homing/1, Scope21/1, Supervisor2/1(homeSwitch)
  Homing_start/1 -> Supervisor2/3(Rotate_ready)
  Product/1 -> Homing Running Switch/1
  Gain/1 -> Saturation1/1
  Saturation1/1 -> Motor X [Nm]/1
  Constant1/1 -> Homing Running Switch1/3
  Homing Running Switch1/1 -> quintic trajectory time/1
  Constant2/1 -> quintic trajectory time/2
  Constant3/1 -> quintic trajectory time/3
  quintic trajectory time/1 -> Sum/2, Supervisor2/4(toPoint_traject), Scope/1
  Supervisor2/5(freddy) -> Unit Delay/1
  Unit Delay/1 -> Homing Running Switch1/2

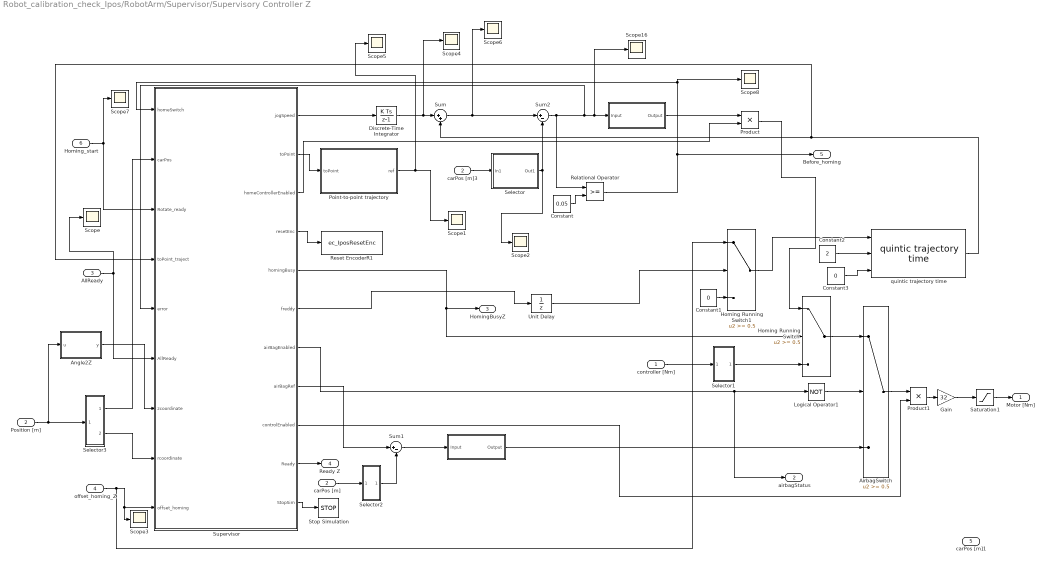
== system Robot_calibration_check_Ipos/RobotArm/Supervisor/Supervisory Controller Z ==
  controller [Nm] : Inport
  carPos [m] : Inport  Port=2
  AllReady : Inport  Port=3
  offset_homing_Z : Inport  Port=4
  carPos [m]1 : Inport  Port=5
  Homing_start : Inport  Port=6
  "    " : Subsystem
  "     " : Subsystem
  AirbagSwitch : Switch  Threshold=0.5
  Angle2Z : MATLAB Function  TreatAsAtomicUnit=on
  Constant : Constant  Value=0.05
  Constant1 : Constant  Value=0
  Constant2 : Constant  Value=2
  Constant3 : Constant  Value=0
  Discrete-Time Integrator : DiscreteIntegrator  SampleTime=-1  ICPrevOutput=DiscIntNeverNeededParam  ICPrevScaledInput=DiscIntNeverNeededParam
  Gain : Gain  Gain=32
  Homing Running Switch : Switch  Threshold=0.5
  Homing Running Switch1 : Switch  Threshold=0.5
  Logical Operator1 : Logic  Operator=NOT  AllPortsSameDT=off  OutDataTypeStr=boolean
  Point-to-point trajectory : Subsystem
  Position [m] : InportShadow  Port=2
  Product : Product  RndMeth=Zero
  Product1 : Product  RndMeth=Zero
  Relational Operator : RelationalOperator  OutDataTypeStr=boolean  RndMeth=Nearest
  Reset EncoderR1 : S-Function  FunctionName=ec_IposResetEnc  Parameters=ipos_id  SFunctionDeploymentMode=off  EnableBusSupport=off  mask{ipos_id=2}
      mask prompts: ipos_id "Ipos ID (from 0 till 3)"
  Saturation1 : Saturate  UpperLimit=127  LowerLimit=-127
  Scope{,1..8,16} (10 alike) : Scope
  Selector : Subsystem
  Selector1 : Subsystem
  Selector2 : Subsystem
  Selector3 : Subsystem
  Stop Simulation : Stop
  Sum : Sum  Inputs=|++
  Sum1 : Sum  Inputs=|+-
  Sum2 : Sum  Inputs=|+-
  Supervisor : Stateflow chart  TreatAsAtomicUnit=on
  Unit Delay : UnitDelay  SampleTime=-1  HasFrameUpgradeWarning=on
  carPos [m]3 : InportShadow  Port=2
  quintic trajectory time : Quintic_Polynomial_Trajectory_Library/quintic trajectory time  SystemSampleTime=-1  VariantActivationTime=update diagram  Latency=0  AutoFrameSizeCalculation=off
      settings: SourceProductName=Robotarm library
  Motor [Nm] : Outport
  airbagStatus : Outport  Port=2
  HomingBusyZ : Outport  Port=3
  Ready Z : Outport  Port=4
  Before_homing : Outport  Port=5
  wires:
  Homing Running Switch/1 -> AirbagSwitch/1
  carPos [m]3/1 -> Selector/1(In1)
  Sum2/1 -> Supervisor/5(error), Scope16/1, "    "/1(Input), Relational Operator/1
  Point-to-point trajectory/1(ref) -> Scope5/1, Scope1/1
  Supervisor/5(homingBusy) -> Homing Running Switch/2, HomingBusyZ/1
  Supervisor/3(homeControllerEnabled) -> Product/2
  Supervisor/2(toPoint) -> Point-to-point trajectory/1(toPoint)
  Supervisor/4(resetEnc) -> Reset EncoderR1/1
  Logical Operator1/1 -> AirbagSwitch/2
  Sum1/1 -> "     "/1(Input)
  carPos [m]/1 -> Selector2/1(In1)
  Supervisor/8(airBagRef) -> Sum1/1
  AirbagSwitch/1 -> Product1/1
  Product1/1 -> Gain/1
  Supervisor/9(controlEnabled) -> Product1/2
  Supervisor/7(airBagEnabled) -> airbagStatus/1, Logical Operator1/1
  Position [m]/1 -> Angle2Z/1(u), Selector3/1(In1)
  Selector/1(Out1) -> Sum2/2, Scope2/1
  Selector1/1(Out1) -> Homing Running Switch/3
  Selector2/1(Out1) -> Sum1/2
  Constant/1 -> Relational Operator/2
  Relational Operator/1 -> Before_homing/1, Scope8/1, Supervisor/1(homeSwitch)
  "     "/1(Output) -> AirbagSwitch/3
  Selector3/1(Out1) -> Supervisor/2(carPos)
  AllReady/1 -> Scope/1, Supervisor/6(AllReady)
  Supervisor/10(Ready) -> Ready Z/1
  Supervisor/11(StopSim) -> Stop Simulation/1
  Angle2Z/1(y) -> Supervisor/7(zcoordinate)
  Selector3/2(Out2) -> Supervisor/8(rcoordinate)
  "    "/1(Output) -> Product/1
  Sum/1 -> Scope6/1, Sum2/1
  Discrete-Time Integrator/1 -> Scope4/1, Sum/1
  offset_homing_Z/1 -> Homing Running Switch1/1, Scope3/1, Supervisor/9(offset_homing)
  Supervisor/1(jogSpeed) -> Discrete-Time Integrator/1
  Homing_start/1 -> Scope7/1, Supervisor/3(Rotate_ready)
  Product/1 -> Homing Running Switch/1
  controller [Nm]/1 -> Selector1/1(controller [Nm])
  Gain/1 -> Saturation1/1
  Saturation1/1 -> Motor [Nm]/1
  Supervisor/6(freddy) -> Unit Delay/1
  Unit Delay/1 -> Homing Running Switch1/2
  Constant1/1 -> Homing Running Switch1/3
  Homing Running Switch1/1 -> quintic trajectory time/1
  Constant2/1 -> quintic trajectory time/2
  Constant3/1 -> quintic trajectory time/3
  quintic trajectory time/1 -> Supervisor/4(toPoint_traject), Sum/2

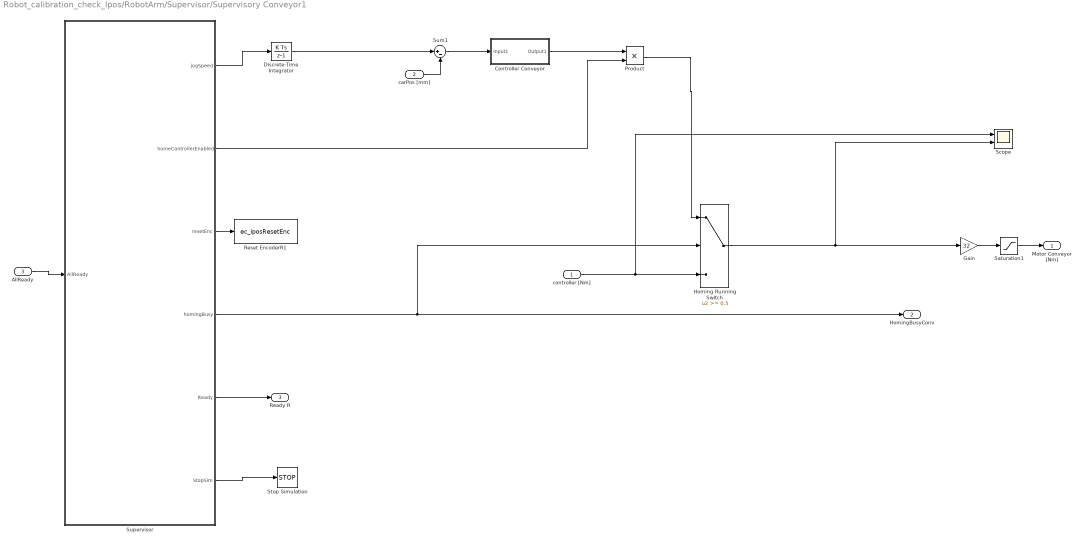
== system Robot_calibration_check_Ipos/RobotArm/Supervisor/Supervisory Conveyor1 ==
  controller [Nm] : Inport
  carPos [mm] : Inport  Port=2
  AllReady : Inport  Port=3
  Controller Conveyor : Subsystem
  Discrete-Time Integrator : DiscreteIntegrator  SampleTime=-1  ICPrevOutput=DiscIntNeverNeededParam  ICPrevScaledInput=DiscIntNeverNeededParam
  Gain : Gain  Gain=32
  Homing Running Switch : Switch  Threshold=0.5
  Product : Product  RndMeth=Zero
  Reset EncoderR1 : S-Function  FunctionName=ec_IposResetEnc  Parameters=ipos_id  SFunctionDeploymentMode=off  EnableBusSupport=off  mask{ipos_id=0}
      mask prompts: ipos_id "Ipos ID (from 0 till 3)"
  Saturation1 : Saturate  UpperLimit=127  LowerLimit=-127
  Scope : Scope  NumInputPorts=2
  Stop Simulation : Stop
  Sum1 : Sum  Inputs=|+-
  Supervisor : Stateflow chart  TreatAsAtomicUnit=on
  Motor Conveyor [Nm] : Outport
  HomingBusyConv : Outport  Port=2
  Ready R : Outport  Port=3
  wires:
  Supervisor/1(jogSpeed) -> Discrete-Time Integrator/1
  Supervisor/4(homingBusy) -> Homing Running Switch/2, HomingBusyConv/1
  Supervisor/2(homeControllerEnabled) -> Product/2
  Supervisor/3(resetEnc) -> Reset EncoderR1/1
  controller [Nm]/1 -> Scope/1, Homing Running Switch/3
  Supervisor/5(Ready) -> Ready R/1
  AllReady/1 -> Supervisor/1(AllReady)
  Supervisor/6(StopSim) -> Stop Simulation/1
  Discrete-Time Integrator/1 -> Sum1/1
  carPos [mm]/1 -> Sum1/2
  Product/1 -> Homing Running Switch/1
  Sum1/1 -> Controller Conveyor/1(Input1)
  Controller Conveyor/1(Output1) -> Product/1
  Homing Running Switch/1 -> Gain/1, Scope/2
  Gain/1 -> Saturation1/1
  Saturation1/1 -> Motor Conveyor [Nm]/1

== system Robot_calibration_check_Ipos/RobotArm/Supervisor/Subsystem/LED Ring ==
  U : Inport
  Subsystem : Subsystem
  Subsystem3 : Subsystem
  wires:
  U/1 -> Subsystem/1(U), Subsystem3/1(In1)
  Subsystem/1(Y) -> Subsystem3/Enable

== system Robot_calibration_check_Ipos/RobotArm/Supervisor/Supervisory Controller R/  ==
  Input : Inport
  Dct1lowpass : sperte_lib/Dct1lowpass  f_den=100
      settings: SourceProductName=SPERTE project library
  Dctintegrator : sperte_lib/Dctintegrator  f_num=0.5
      settings: SourceProductName=SPERTE project library
  Dctleadlag : sperte_lib/Dctleadlag  f_num=6.6667  f_den=60
      settings: SourceProductName=SPERTE project library
  Gain : Gain  Gain=25
  Output : Outport
  wires:
  Dctleadlag/1 -> Dct1lowpass/1
  Dctintegrator/1 -> Dctleadlag/1
  Input/1 -> Gain/1
  Gain/1 -> Dctintegrator/1
  Dct1lowpass/1 -> Output/1

== system Robot_calibration_check_Ipos/RobotArm/Supervisor/Supervisory Controller R/    ==
  Input : Inport
  Dct1lowpass : sperte_lib/Dct1lowpass  f_den=100
      settings: SourceProductName=SPERTE project library
  Dctleadlag : sperte_lib/Dctleadlag  f_num=6.6667  f_den=60
      settings: SourceProductName=SPERTE project library
  Gain : Gain  Gain=25
  Output : Outport
  wires:
  Gain/1 -> Dctleadlag/1
  Dctleadlag/1 -> Dct1lowpass/1
  Dct1lowpass/1 -> Output/1
  Input/1 -> Gain/1

== system Robot_calibration_check_Ipos/RobotArm/Supervisor/Supervisory Controller R/Point-to-point trajectory ==
  toPoint : Inport
  Constant1 : Constant  Value=0
  Discrete Derivative : simulink/Discrete/Discrete Derivative  gainval=1.0  ICPrevScaledInput=0.0  OutMin=[]  OutMax=[]  OutDataType=fixdt(1, 16)  OutScaling=2^-10  DoSatur=off
  Discrete-Time Integrator : DiscreteIntegrator  InitialConditionSource=external  SampleTime=-1  ICPrevOutput=DiscIntNeverNeededParam  ICPrevScaledInput=DiscIntNeverNeededParam
  Limit Acceleration : RateLimiter  RisingSlewLimit=0.8  FallingSlewLimit=-0.8  SampleTimeMode=inherited
  Limit Speed : RateLimiter  RisingSlewLimit=0.6  FallingSlewLimit=-0.6  SampleTimeMode=inherited
  Sum : Sum  Inputs=|++
  ref : Outport
  wires:
  Sum/1 -> Limit Speed/1
  Constant1/1 -> Sum/2, Discrete-Time Integrator/2
  Limit Acceleration/1 -> Discrete-Time Integrator/1
  Discrete Derivative/1 -> Limit Acceleration/1
  Limit Speed/1 -> Discrete Derivative/1
  toPoint/1 -> Sum/1
  Discrete-Time Integrator/1 -> ref/1

== system Robot_calibration_check_Ipos/RobotArm/Supervisor/Supervisory Controller R/Selector1 ==
  controller [Nm] : Inport
  Demux2 : Demux  Outputs=3
  Scope : Scope
  Terminator4 : Terminator
  Terminator5 : Terminator
  Out1 : Outport
  wires:
  Demux2/2 -> Terminator4/1
  controller [Nm]/1 -> Demux2/1
  Demux2/1 -> Scope/1, Out1/1
  Demux2/3 -> Terminator5/1

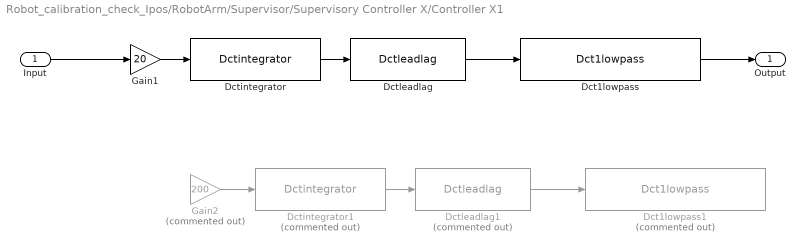
== system Robot_calibration_check_Ipos/RobotArm/Supervisor/Supervisory Controller X/Controller X1 ==
  Input : Inport
  Dct1lowpass : sperte_lib/Dct1lowpass  f_den=200
      settings: SourceProductName=SPERTE project library
  Dct1lowpass1 : sperte_lib/Dct1lowpass  Commented=on  f_den=200
      settings: SourceProductName=SPERTE project library
  Dctintegrator : sperte_lib/Dctintegrator  f_num=0.5
      settings: SourceProductName=SPERTE project library
  Dctintegrator1 : sperte_lib/Dctintegrator  Commented=on  f_num=0.5
      settings: SourceProductName=SPERTE project library
  Dctleadlag : sperte_lib/Dctleadlag  f_num=10  f_den=90
      settings: SourceProductName=SPERTE project library
  Dctleadlag1 : sperte_lib/Dctleadlag  Commented=on  f_num=10  f_den=90
      settings: SourceProductName=SPERTE project library
  Gain1 : Gain  Gain=20
  Gain2 : Gain  Commented=on  Gain=200
  Output : Outport
  wires:
  Dctleadlag/1 -> Dct1lowpass/1
  Dctintegrator/1 -> Dctleadlag/1
  Gain1/1 -> Dctintegrator/1
  Dctleadlag1/1 -> Dct1lowpass1/1
  Gain2/1 -> Dctintegrator1/1
  Dctintegrator1/1 -> Dctleadlag1/1
  Dct1lowpass/1 -> Output/1
  Input/1 -> Gain1/1

== system Robot_calibration_check_Ipos/RobotArm/Supervisor/Supervisory Controller X/Controller X2 ==
  Input : Inport
  Dct1lowpass : sperte_lib/Dct1lowpass  f_den=200
      settings: SourceProductName=SPERTE project library
  Dctleadlag : sperte_lib/Dctleadlag  f_num=10  f_den=90
      settings: SourceProductName=SPERTE project library
  Gain1 : Gain  Gain=20
  Output : Outport
  wires:
  Gain1/1 -> Dctleadlag/1
  Input/1 -> Gain1/1
  Dctleadlag/1 -> Dct1lowpass/1
  Dct1lowpass/1 -> Output/1

== system Robot_calibration_check_Ipos/RobotArm/Supervisor/Supervisory Controller X/Point-to-point trajectory ==
  toPoint : Inport
  Constant1 : Constant  Value=0
  Discrete Derivative : simulink/Discrete/Discrete Derivative  gainval=1.0  ICPrevScaledInput=0.0  OutMin=[]  OutMax=[]  OutDataType=fixdt(1, 16)  OutScaling=2^-10  DoSatur=off
  Discrete-Time Integrator : DiscreteIntegrator  InitialConditionSource=external  SampleTime=-1  ICPrevOutput=DiscIntNeverNeededParam  ICPrevScaledInput=DiscIntNeverNeededParam
  Limit Acceleration : RateLimiter  RisingSlewLimit=0.5  FallingSlewLimit=-0.5  SampleTimeMode=inherited
  Limit Speed : RateLimiter  RisingSlewLimit=0.4  FallingSlewLimit=-0.4  SampleTimeMode=inherited
  Sum : Sum  Inputs=|++
  ref : Outport
  wires:
  Discrete-Time Integrator/1 -> ref/1
  toPoint/1 -> Sum/1
  Limit Speed/1 -> Discrete Derivative/1
  Discrete Derivative/1 -> Limit Acceleration/1
  Limit Acceleration/1 -> Discrete-Time Integrator/1
  Constant1/1 -> Discrete-Time Integrator/2, Sum/2
  Sum/1 -> Limit Speed/1

== system Robot_calibration_check_Ipos/RobotArm/Supervisor/Supervisory Controller X/Selector ==
  controller [Nm] : Inport
  Demux2 : Demux  Outputs=3
  Terminator4 : Terminator
  Terminator5 : Terminator
  Out1 : Outport
  wires:
  Demux2/3 -> Terminator5/1
  Demux2/1 -> Terminator4/1
  controller [Nm]/1 -> Demux2/1
  Demux2/2 -> Out1/1

== system Robot_calibration_check_Ipos/RobotArm/Supervisor/Supervisory Controller X/Selector1 ==
  In1 : Inport
  Demux2 : Demux  Outputs=3
  Terminator4 : Terminator
  Terminator5 : Terminator
  Out1 : Outport
  wires:
  Demux2/2 -> Out1/1
  In1/1 -> Demux2/1
  Demux2/1 -> Terminator4/1
  Demux2/3 -> Terminator5/1

== system Robot_calibration_check_Ipos/RobotArm/Supervisor/Supervisory Controller X/Selector2 ==
  In1 : Inport
  Demux2 : Demux  Outputs=3
  Terminator4 : Terminator
  Terminator5 : Terminator
  Out1 : Outport
  wires:
  Demux2/2 -> Out1/1
  In1/1 -> Demux2/1
  Demux2/1 -> Terminator4/1
  Demux2/3 -> Terminator5/1

== system Robot_calibration_check_Ipos/RobotArm/Supervisor/Supervisory Controller X/Selector3 ==
  In1 : Inport
  Demux2 : Demux  Outputs=3
  Terminator4 : Terminator
  Terminator5 : Terminator
  carPos : Outport
  wires:
  Demux2/3 -> Terminator5/1
  Demux2/1 -> Terminator4/1
  In1/1 -> Demux2/1
  Demux2/2 -> carPos/1

== system Robot_calibration_check_Ipos/RobotArm/Supervisor/Supervisory Controller Z/     ==
  Input : Inport
  Dct1lowpass : sperte_lib/Dct1lowpass  f_den=200
      settings: SourceProductName=SPERTE project library
  Dctintegrator : sperte_lib/Dctintegrator  f_num=0.5
      settings: SourceProductName=SPERTE project library
  Dctleadlag : sperte_lib/Dctleadlag  f_num=10  f_den=90
      settings: SourceProductName=SPERTE project library
  Gain : Gain  Gain=20
  Output : Outport
  wires:
  Gain/1 -> Dctintegrator/1
  Dct1lowpass/1 -> Output/1
  Dctleadlag/1 -> Dct1lowpass/1
  Dctintegrator/1 -> Dctleadlag/1
  Input/1 -> Gain/1

== system Robot_calibration_check_Ipos/RobotArm/Supervisor/Supervisory Controller Z/      ==
  Input : Inport
  Dct1lowpass : sperte_lib/Dct1lowpass  f_den=200
      settings: SourceProductName=SPERTE project library
  Dctleadlag : sperte_lib/Dctleadlag  f_num=10  f_den=90
      settings: SourceProductName=SPERTE project library
  Gain : Gain  Gain=30
  Output : Outport
  wires:
  Gain/1 -> Dctleadlag/1
  Dctleadlag/1 -> Dct1lowpass/1
  Dct1lowpass/1 -> Output/1
  Input/1 -> Gain/1

== system Robot_calibration_check_Ipos/RobotArm/Supervisor/Supervisory Controller Z/Point-to-point trajectory ==
  toPoint : Inport
  Constant1 : Constant  Value=0
  Discrete Derivative : simulink/Discrete/Discrete Derivative  gainval=1.0  ICPrevScaledInput=0.0  OutMin=[]  OutMax=[]  OutDataType=fixdt(1, 16)  OutScaling=2^-10  DoSatur=off
  Discrete-Time Integrator : DiscreteIntegrator  InitialConditionSource=external  SampleTime=-1  ICPrevOutput=DiscIntNeverNeededParam  ICPrevScaledInput=DiscIntNeverNeededParam
  Limit Acceleration : RateLimiter  RisingSlewLimit=0.5  FallingSlewLimit=-0.5  SampleTimeMode=inherited
  Limit Speed : RateLimiter  RisingSlewLimit=0.2  FallingSlewLimit=-0.2  SampleTimeMode=inherited
  Sum : Sum  Inputs=|++
  ref : Outport
  wires:
  Sum/1 -> Limit Speed/1
  Constant1/1 -> Sum/2, Discrete-Time Integrator/2
  Limit Acceleration/1 -> Discrete-Time Integrator/1
  Discrete Derivative/1 -> Limit Acceleration/1
  Limit Speed/1 -> Discrete Derivative/1
  toPoint/1 -> Sum/1
  Discrete-Time Integrator/1 -> ref/1

== system Robot_calibration_check_Ipos/RobotArm/Supervisor/Supervisory Controller Z/Selector ==
  In1 : Inport
  Demux2 : Demux  Outputs=3
  Terminator4 : Terminator
  Terminator5 : Terminator
  Out1 : Outport
  wires:
  Demux2/1 -> Terminator4/1
  In1/1 -> Demux2/1
  Demux2/2 -> Terminator5/1
  Demux2/3 -> Out1/1

== system Robot_calibration_check_Ipos/RobotArm/Supervisor/Supervisory Controller Z/Selector1 ==
  controller [Nm] : Inport
  Demux2 : Demux  Outputs=3
  Terminator4 : Terminator
  Terminator5 : Terminator
  Out1 : Outport
  wires:
  Demux2/3 -> Out1/1
  Demux2/2 -> Terminator5/1
  controller [Nm]/1 -> Demux2/1
  Demux2/1 -> Terminator4/1

== system Robot_calibration_check_Ipos/RobotArm/Supervisor/Supervisory Controller Z/Selector2 ==
  In1 : Inport
  Demux2 : Demux  Outputs=3
  Terminator4 : Terminator
  Terminator5 : Terminator
  Out1 : Outport
  wires:
  Demux2/1 -> Terminator4/1
  In1/1 -> Demux2/1
  Demux2/2 -> Terminator5/1
  Demux2/3 -> Out1/1

== system Robot_calibration_check_Ipos/RobotArm/Supervisor/Supervisory Controller Z/Selector3 ==
  In1 : Inport
  Demux2 : Demux  Outputs=3
  Terminator5 : Terminator
  Out1 : Outport
  Out2 : Outport  Port=2
  wires:
  Demux2/3 -> Out1/1
  Demux2/2 -> Terminator5/1
  In1/1 -> Demux2/1
  Demux2/1 -> Out2/1
